simulink model "EV2"  (R2021a)
settings: Solver=ode4  StartTime=0.0  StopTime=5000  FixedStep=0.01  RelTol=1e-4
model workspace (MAT data in the model file):
  Bcapacity = 70
  J = 300
  Km = 10
  R = 0.7
  Rint = 1.8
  SOCinit = 0.8
  V0 = 300
  airFrictionCoefficient = 0.2
  gearRatio = 1.5
  m = 800
  motL = 0.2
  motR = 4
  socInit = 0.8
  tireResistance = 5
settings Model: OrderedModelArguments=off  Creator=himi  LastModifiedBy=himi
settings SolverCC: AlgebraicLoopSolver=TrustRegion
settings DebuggingCC: SFMachineParentedDataDiag=warning

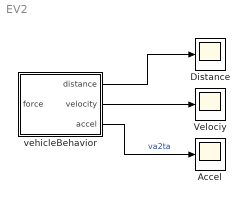
== system EV2 ==
  Accel : Scope
  Distance : Scope
  Velociy : Scope
  vehicleBehavior : Subsystem
  wires:
  vehicleBehavior/2(velocity) -> Velociy/1
  vehicleBehavior/1(distance) -> Distance/1
  vehicleBehavior/3(accel) -> Accel/1  "va2ta"

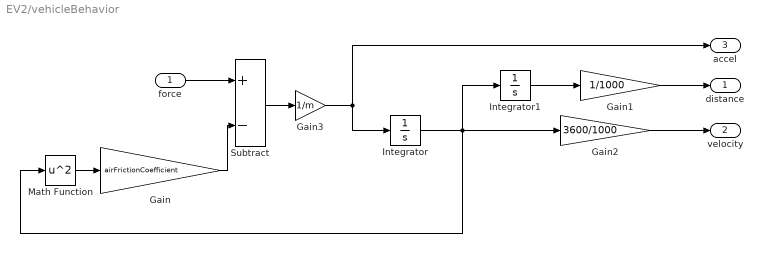
== system EV2/vehicleBehavior ==
  force : Inport
  Gain : Gain  Gain=airFrictionCoefficient
  Gain1 : Gain  Gain=1/1000
  Gain2 : Gain  Gain=3600/1000
  Gain3 : Gain  Gain=1/m
  Integrator : Integrator
  Integrator1 : Integrator
  Math Function : Math  Operator=square  SaturateOnIntegerOverflow=on
  Subtract : Sum  Inputs=+-
  distance : Outport
  velocity : Outport  Port=2
  accel : Outport  Port=3
  wires:
  Gain3/1 -> Integrator/1, accel/1
  force/1 -> Subtract/1
  Integrator/1 -> Integrator1/1, Gain2/1, Math Function/1
  Integrator1/1 -> Gain1/1
  Subtract/1 -> Gain3/1
  Math Function/1 -> Gain/1
  Gain/1 -> Subtract/2
  Gain1/1 -> distance/1
  Gain2/1 -> velocity/1
